simulink model "Model_v13"  (R2019a)
settings: Solver=VariableStepAuto  StartTime=0.0  StopTime=t_sim  MaxStep=1e-3  RelTol=1e-6
values from neighbouring files (symbols this model uses):
  b_wheel = 5e-4    (= 0.0005)    [Parameters.m]    (also in UKFMeasurementFcn.m; UKFTransitionFcn.m)
  H = 0.075    [Parameters.m]    (also in SMC_one_wheel.m; UKFMeasurementFcn.m; UKFTransitionFcn.m)
  J = 0.001    [Parameters.m]    (also in SMC_one_wheel.m = 0.00015; UKFMeasurementFcn.m; UKFTransitionFcn.m)
  Km = 36.9e-3    (= 0.0369)    [Parameters.m]    (also in SMC_one_wheel.m; UKFMeasurementFcn.m; UKFTransitionFcn.m)
  l = l_front + l_rear    (= 0.401)    [Parameters.m]    (also in SMC_one_wheel.m; UKFMeasurementFcn.m; UKFTransitionFcn.m)
  l_front = 0.1968    [Parameters.m]    (also in SMC_one_wheel.m; UKFMeasurementFcn.m; UKFTransitionFcn.m)
  l_rear = 0.2042    [Parameters.m]    (also in SMC_one_wheel.m; UKFMeasurementFcn.m; UKFTransitionFcn.m)
  Lm = 0.463e-3    (= 0.000463)    [Parameters.m]    (also in SMC_one_wheel.m; UKFMeasurementFcn.m; UKFTransitionFcn.m)
  M = 3.832    [Parameters.m]    (also in SMC_one_wheel.m = 0.958; UKFMeasurementFcn.m; UKFTransitionFcn.m)
  R = 0.055    [Parameters.m]    (also in SMC_one_wheel.m; UKFMeasurementFcn.m; UKFTransitionFcn.m; slip_rate.m = args(3))
  Rm = 0.608    [Parameters.m]    (also in SMC_one_wheel.m; UKFMeasurementFcn.m; UKFTransitionFcn.m)
  t_dec = 5    [Parameters.m]
  V_0 = 1    [Parameters.m]
  V_max = 24    [Parameters.m]
  W = M*g    (= 37.59192)    [Parameters.m]    (also in SMC_one_wheel.m = 9.39798; UKFMeasurementFcn.m; UKFTransitionFcn.m)
  w_0 = (1-slip)*V_0/R    (= 18.1818181818)    [Parameters.m]    (also in SMC_one_wheel.m = 90.9090909091)
  WheelSS_A = [-b_wheel/J, Km/J, 0, 0 ... (first row only)    [Parameters.m]
  WheelSS_B = [-R/J, 0, 0, 0 ... (first row only)    [Parameters.m]
  WheelSS_C = [1, 0, 0, 0 ... (first row only)    [Parameters.m]
  WheelSS_D = [0, 0, 0, 0 ... (first row only)    [Parameters.m]
  WheelSS_ICs = [w_0, 0, w_0, 0]    [Parameters.m]
undefined symbols (not defined in the file or in its folder): Discrete, Time
libraries: simulink x11, eeGeneralControl x2, ctrlSharedLib x2
settings Model: Creator=Iansweeney  LastModifiedBy=Iansweeney
settings DataIOCC: ReturnWorkspaceOutputs=off
settings DebuggingCC: UnderSpecifiedDimensionMsg=warning  ArithmeticOperatorsInVariantConditions=warning

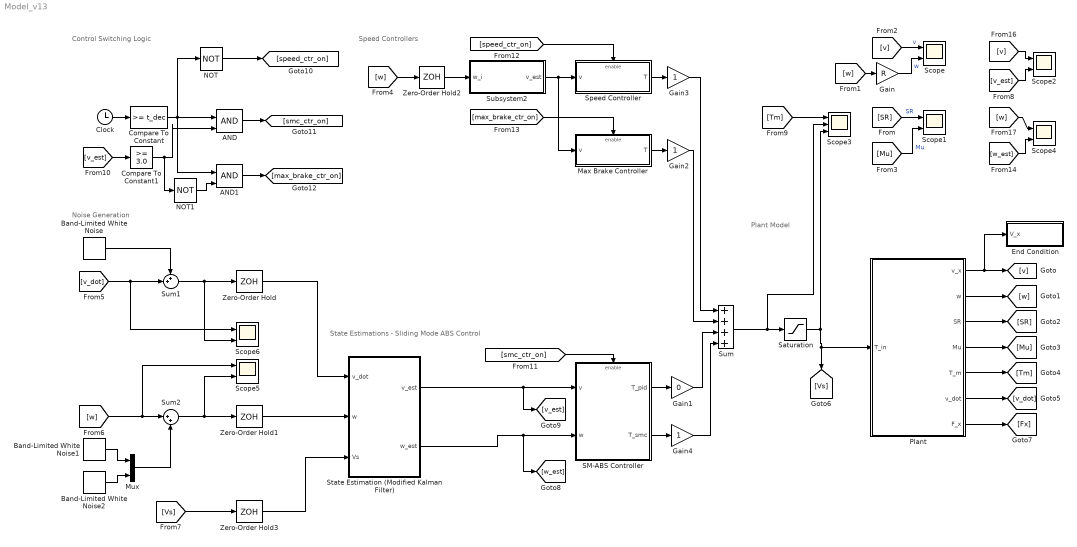
== system Model_v13 ==
  note: State Estimations - Sliding Mode ABS Control
  note: Noise Generation
  note: Speed Controllers
  note: Plant Model
  note: Control Switching Logic
  AND : Logic  IconShape=distinctive  AllPortsSameDT=off  OutDataTypeStr=boolean
  AND1 : Logic  IconShape=distinctive  AllPortsSameDT=off  OutDataTypeStr=boolean
  Band-Limited White Noise : simulink/Sources/Band-Limited White Noise  Cov=[0.001]  Ts=0.001  seed=[23341]
  Band-Limited White Noise1 : simulink/Sources/Band-Limited White Noise  Cov=[0.01]  Ts=0.001  seed=[11111]
  Band-Limited White Noise2 : simulink/Sources/Band-Limited White Noise  Cov=[0.01]  Ts=0.001  seed=[22222]
  Clock : Clock
  Compare To Constant : simulink/Logic and Bit Operations/Compare To Constant  relop=>=  const=t_dec  OutDataTypeStr=boolean
  Compare To Constant1 : simulink/Logic and Bit Operations/Compare To Constant  relop=>=  const=3.0  OutDataTypeStr=boolean
  End Condition : Subsystem
  Gain : Gain  Gain=R
  Gain1 : Gain  Gain=0
  Gain2 : Gain
  Gain3 : Gain
  Gain4 : Gain
  Max Brake Controller : Subsystem
  Mux : Mux  Inputs=2
  NOT : Logic  Operator=NOT  IconShape=distinctive  AllPortsSameDT=off  OutDataTypeStr=boolean
  NOT1 : Logic  Operator=NOT  IconShape=distinctive  AllPortsSameDT=off  OutDataTypeStr=boolean
  Plant : Subsystem
  SM-ABS Controller : Subsystem  TreatAsAtomicUnit=on
  Saturation : Saturate  UpperLimit=V_max  LowerLimit=-V_max
  Scope{,1..2,4..6} (6 alike) : Scope  NumInputPorts=2
  Scope3 : Scope  NumInputPorts=3
  Speed Controller : Subsystem
  State Estimation (Modified Kalman Filter) : Subsystem
  Subsystem2 : Subsystem
  Sum : Sum  Inputs=++++
  Sum1 : Sum  Inputs=++|
  Sum2 : Sum  Inputs=|++
  Zero-Order Hold{,1..3} (4 alike) : ZeroOrderHold  SampleTime=0.01
  wires:
  Plant/1(v_x) -> End Condition/1(V_x), [v]
  Plant/2(w) -> [w]
  Plant/3(SR) -> [SR]
  Plant/4(Mu) -> [Mu]
  Gain/1 -> Scope/2  "w"
  [SR] -> Scope1/1  "SR"
  [w] -> Gain/1
  [v] -> Scope/1  "v"
  [Mu] -> Scope1/2  "Mu"
  Saturation/1 -> Scope3/3, Plant/1(T_in), [Vs]
  Sum/1 -> Scope3/2, Saturation/1
  Plant/5(T_m) -> [Tm]
  [Tm] -> Scope3/1
  SM-ABS Controller/1(T_pid) -> Gain1/1
  Gain1/1 -> Sum/3
  Speed Controller/1(T) -> Gain3/1
  Gain3/1 -> Sum/1
  SM-ABS Controller/2(T_smc) -> Gain4/1
  Gain4/1 -> Sum/4
  Plant/6(v_dot) -> [v_dot]
  Subsystem2/1(v_est) -> Max Brake Controller/1(v), Speed Controller/1(v)
  [w] -> Zero-Order Hold2/1
  Zero-Order Hold2/1 -> Subsystem2/1(w_i)
  Zero-Order Hold/1 -> State Estimation (Modified Kalman Filter)/1(v_dot)
  [Vs] -> Zero-Order Hold3/1
  Zero-Order Hold3/1 -> State Estimation (Modified Kalman Filter)/3(Vs)
  Zero-Order Hold1/1 -> State Estimation (Modified Kalman Filter)/2(w)
  State Estimation (Modified Kalman Filter)/1(v_est) -> [v_est], SM-ABS Controller/1(v)
  Plant/7(F_x) -> [Fx]
  State Estimation (Modified Kalman Filter)/2(w_est) -> [w_est], SM-ABS Controller/2(w)
  [v_est] -> Scope2/2
  [v] -> Scope2/1
  [w] -> Scope4/1
  [w_est] -> Scope4/2
  Band-Limited White Noise/1 -> Sum1/1
  Band-Limited White Noise1/1 -> Mux/1
  Mux/1 -> Sum2/2
  [w] -> Scope5/1, Sum2/1
  Sum2/1 -> Scope5/2, Zero-Order Hold1/1
  [v_dot] -> Scope6/1, Sum1/2
  Sum1/1 -> Scope6/2, Zero-Order Hold/1
  Clock/1 -> Compare To Constant/1
  [v_est] -> Compare To Constant1/1
  AND/1 -> [smc_ctr_on]
  Compare To Constant/1 -> AND1/1, NOT/1, AND/1
  Compare To Constant1/1 -> NOT1/1, AND/2
  [smc_ctr_on] -> SM-ABS Controller/Enable
  NOT/1 -> [speed_ctr_on]
  [speed_ctr_on] -> Speed Controller/Enable
  NOT1/1 -> AND1/2
  AND1/1 -> [max_brake_ctr_on]
  Gain2/1 -> Sum/2
  Max Brake Controller/1(T) -> Gain2/1
  [max_brake_ctr_on] -> Max Brake Controller/Enable
  Band-Limited White Noise2/1 -> Mux/2

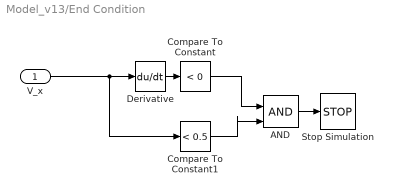
== system Model_v13/End Condition ==
  V_x : Inport
  AND : Logic  IconShape=distinctive  AllPortsSameDT=off  OutDataTypeStr=boolean
  Compare To Constant : simulink/Logic and Bit Operations/Compare To Constant  relop=<  const=0  OutDataTypeStr=boolean
  Compare To Constant1 : simulink/Logic and Bit Operations/Compare To Constant  relop=<  const=0.5  OutDataTypeStr=boolean
  Derivative : Derivative
  Stop Simulation : Stop
  wires:
  AND/1 -> Stop Simulation/1
  Derivative/1 -> Compare To Constant/1
  Compare To Constant/1 -> AND/1
  Compare To Constant1/1 -> AND/2
  V_x/1 -> Compare To Constant1/1, Derivative/1

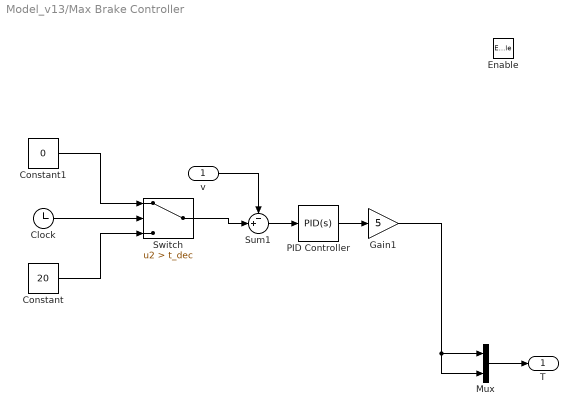
== system Model_v13/Max Brake Controller ==
  v : Inport
  Enable : EnablePort
  Clock : Clock
  Constant : Constant  Value=20
  Constant1 : Constant  Value=0
  Gain1 : Gain  Gain=5
  Mux : Mux  Inputs=2
  PID Controller : simulink/Continuous/PID Controller  Controller=PID  Form=Parallel  TimeDomain=Continuous-time  SampleTime=-1  IntegratorMethod=Forward Euler  FilterMethod=Forward Euler  ControllerParametersSource=internal  P=1  I=0  D=0  UseFilter=on  N=100  TunerSelectOption=Transfer Function Based (PID Tuner App)  InitialConditionSource=internal  InitialConditionForIntegrator=0  InitialConditionForFilter=0  DifferentiatorICPrevScaledInput=0  ExternalReset=none  TrackingMode=off  Kt=1  LimitOutput=off  UpperSaturationLimit=inf  LowerSaturationLimit=-inf  LinearizeAsGain=on  AntiWindupMode=none  Kb=1  POutMin=[]  POutMax=[]  IOutMin=[]  IOutMax=[]  DOutMin=[]  DOutMax=[]  NOutMin=[]  NOutMax=[]  SumOutMin=[]  SumOutMax=[]  SaturationOutMin=[]  SaturationOutMax=[]  PParamMin=[]  PParamMax=[]  IParamMin=[]  IParamMax=[]  DParamMin=[]  DParamMax=[]  NParamMin=[]  NParamMax=[]  KbParamMin=[]  KbParamMax=[]  KtParamMin=[]  KtParamMax=[]  KbOutMin=[]  KbOutMax=[]  KtOutMin=[]  KtOutMax=[]  IntegratorOutMin=[]  IntegratorOutMax=[]  FilterOutMin=[]  FilterOutMax=[]  SumI1OutMin=[]  SumI1OutMax=[]  SumI2OutMin=[]  SumI2OutMax=[]  SumI3OutMin=[]  SumI3OutMax=[]  SumI4OutMin=[]  SumI4OutMax=[]  SumDOutMin=[]  SumDOutMax=[]  DifferentiatorOutMin=[]  DifferentiatorOutMax=[]  FilterDiffOutCoefMin=[]  FilterDiffOutCoefMax=[]  ReciprocalOutMin=[]  ReciprocalOutMax=[]  SumDenOutMin=[]  SumDenOutMax=[]  SumNumOutMin=[]  SumNumOutMax=[]  DivideOutMin=[]  DivideOutMax=[]  IntegratorContinuousStateAttributes=''  IntegratorStateMustResolveToSignalObject=off  IntegratorRTWStateStorageClass=Auto  FilterContinuousStateAttributes=''  FilterStateMustResolveToSignalObject=off  FilterRTWStateStorageClass=Auto  ParallelPVariant=InternalParameters  IdealPVariant=Disabled  IVariant=InternalParameters  DVariant=InternalParameters  IntegratorVariant=Continuous  SatVariant=Disabled  AWVariant=Passthrough  PCopyVariant=Disabled  TRVariant=Disabled  FdbkBlocksVariant=Forward  IdealPFdbkVariant=Disabled  SatFdbkVariant=Disabled  DerivativeFilterVariant=ContFilter  NVariant=InternalParameters  NCopyVariant=Disabled  FilterICVariant=InternalICsFilter  IntegratorICVariant=InternalICs  ExternalResetVariant=Disabled  TRSumVariant=Passthrough  SumFdbkVariant=Disabled  SumVariant=Sum_PID
  Sum1 : Sum  Inputs=-+|
  Switch : Switch  Criteria=u2 > Threshold  Threshold=t_dec
  T : Outport  OutputWhenDisabled=reset  InitialOutput=[0, 0]
  wires:
  PID Controller/1 -> Gain1/1
  Switch/1 -> Sum1/2
  Sum1/1 -> PID Controller/1
  Mux/1 -> T/1
  Gain1/1 -> Mux/2, Mux/1
  v/1 -> Sum1/1
  Constant/1 -> Switch/3
  Constant1/1 -> Switch/1
  Clock/1 -> Switch/2

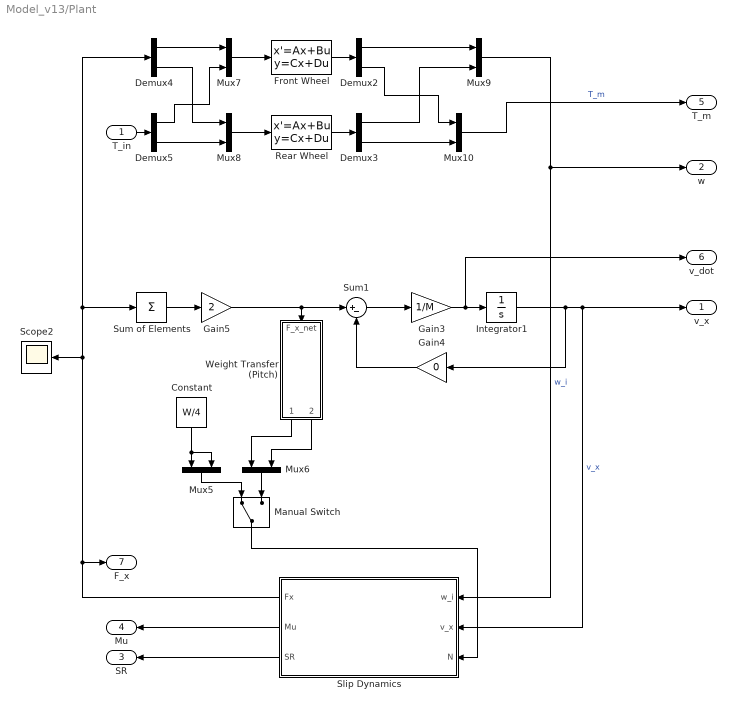
== system Model_v13/Plant ==
  T_in : Inport
  Constant : Constant  Value=W/4
  Demux{2..5} (4 alike) : Demux  Outputs=2
  Front Wheel : StateSpace  A=[-b_wheel/J, Km/J; -Km/J, -Rm/Lm]  B=[-R/J, 0; 0, 1/Lm]  C=[1, 0; 0, Km]  D=[0, 0; 0, 0]  InitialCondition=[w_0, 0]
  Gain3 : Gain  Gain=1/M
  Gain4 : Gain  Gain=0
  Gain5 : Gain  Gain=2
  Integrator1 : Integrator  InitialCondition=V_0
  Manual Switch : ManualSwitch
  Mux{5..10} (6 alike) : Mux  Inputs=2
  Rear Wheel : StateSpace  A=[-b_wheel/J, Km/J; -Km/J, -Rm/Lm]  B=[-R/J, 0; 0, 1/Lm]  C=[1, 0; 0, Km]  D=[0, 0; 0, 0]  InitialCondition=[w_0, 0]
  Scope2 : Scope
  Slip Dynamics : Subsystem
  Sum of Elements : Sum  Inputs=+
  Sum1 : Sum  Inputs=|+-
  Weight Transfer (Pitch) : Subsystem
  v_x : Outport
  w : Outport  Port=2
  SR : Outport  Port=3
  Mu : Outport  Port=4
  T_m : Outport  Port=5
  v_dot : Outport  Port=6
  F_x : Outport  Port=7
  wires:
  Weight Transfer (Pitch)/1(F_z_front) -> Mux6/1
  Weight Transfer (Pitch)/2(F_z_rear) -> Mux6/2
  Gain3/1 -> v_dot/1, Integrator1/1
  Mux5/1 -> Manual Switch/1
  Gain4/1 -> Sum1/2
  T_in/1 -> Demux5/1
  Sum1/1 -> Gain3/1
  Mux6/1 -> Manual Switch/2
  Constant/1 -> Mux5/2, Mux5/1
  Mux9/1 -> w/1, Slip Dynamics/1(w_i)  "w_i"
  Gain5/1 -> Weight Transfer (Pitch)/1(F_x_net), Sum1/1
  Sum of Elements/1 -> Gain5/1
  Integrator1/1 -> Gain4/1, Slip Dynamics/2(v_x), v_x/1  "v_x"
  Mux7/1 -> Front Wheel/1
  Front Wheel/1 -> Demux2/1
  Demux2/1 -> Mux9/1
  Mux8/1 -> Rear Wheel/1
  Rear Wheel/1 -> Demux3/1
  Demux3/1 -> Mux9/2
  Demux4/1 -> Mux7/1
  Demux4/2 -> Mux8/1
  Demux5/1 -> Mux7/2
  Demux5/2 -> Mux8/2
  Demux3/2 -> Mux10/2
  Demux2/2 -> Mux10/1
  Mux10/1 -> T_m/1  "T_m"
  Slip Dynamics/1(Fx) -> F_x/1, Demux4/1, Sum of Elements/1, Scope2/1
  Manual Switch/1 -> Slip Dynamics/3(N)
  Slip Dynamics/2(Mu) -> Mu/1
  Slip Dynamics/3(SR) -> SR/1

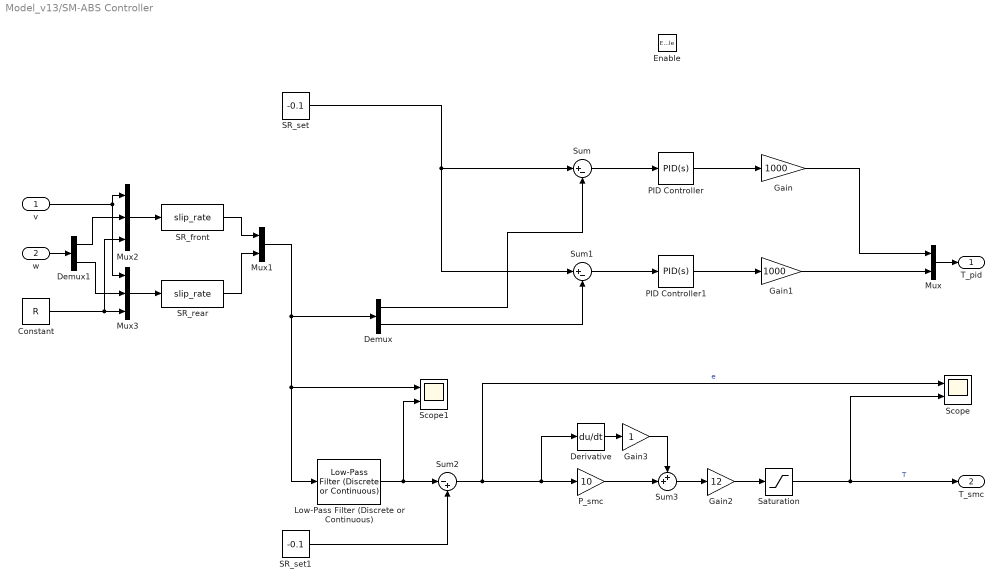
== system Model_v13/SM-ABS Controller ==
  v : Inport
  w : Inport  Port=2
  Enable : EnablePort
  Constant : Constant  Value=R
  Demux : Demux  Outputs=2
  Demux1 : Demux  Outputs=2
  Derivative : Derivative
  Gain : Gain  Gain=1000
  Gain1 : Gain  Gain=1000
  Gain2 : Gain  Gain=12
  Gain3 : Gain
  Low-Pass Filter (Discrete or Continuous) : eeGeneralControl/Low-Pass Filter (Discrete or Continuous)  K=1  T=0.05  B=inf  A=-inf  Ts=-1
      settings: SourceProductName=Simscape Electrical
  Mux : Mux  Inputs=2
  Mux1 : Mux  Inputs=2
  Mux2 : Mux  Inputs=3
  Mux3 : Mux  Inputs=3
  PID Controller : simulink/Continuous/PID Controller  Controller=PID  Form=Parallel  TimeDomain=Continuous-time  SampleTime=-1  IntegratorMethod=Forward Euler  FilterMethod=Forward Euler  ControllerParametersSource=internal  P=1  I=1  D=0  UseFilter=on  N=100  TunerSelectOption=Transfer Function Based (PID Tuner App)  InitialConditionSource=internal  InitialConditionForIntegrator=0  InitialConditionForFilter=0  DifferentiatorICPrevScaledInput=0  ExternalReset=none  TrackingMode=off  Kt=1  LimitOutput=off  UpperSaturationLimit=inf  LowerSaturationLimit=-inf  LinearizeAsGain=on  AntiWindupMode=none  Kb=1  POutMin=[]  POutMax=[]  IOutMin=[]  IOutMax=[]  DOutMin=[]  DOutMax=[]  NOutMin=[]  NOutMax=[]  SumOutMin=[]  SumOutMax=[]  SaturationOutMin=[]  SaturationOutMax=[]  PParamMin=[]  PParamMax=[]  IParamMin=[]  IParamMax=[]  DParamMin=[]  DParamMax=[]  NParamMin=[]  NParamMax=[]  KbParamMin=[]  KbParamMax=[]  KtParamMin=[]  KtParamMax=[]  KbOutMin=[]  KbOutMax=[]  KtOutMin=[]  KtOutMax=[]  IntegratorOutMin=[]  IntegratorOutMax=[]  FilterOutMin=[]  FilterOutMax=[]  SumI1OutMin=[]  SumI1OutMax=[]  SumI2OutMin=[]  SumI2OutMax=[]  SumI3OutMin=[]  SumI3OutMax=[]  SumI4OutMin=[]  SumI4OutMax=[]  SumDOutMin=[]  SumDOutMax=[]  DifferentiatorOutMin=[]  DifferentiatorOutMax=[]  FilterDiffOutCoefMin=[]  FilterDiffOutCoefMax=[]  ReciprocalOutMin=[]  ReciprocalOutMax=[]  SumDenOutMin=[]  SumDenOutMax=[]  SumNumOutMin=[]  SumNumOutMax=[]  DivideOutMin=[]  DivideOutMax=[]  IntegratorContinuousStateAttributes=''  IntegratorStateMustResolveToSignalObject=off  IntegratorRTWStateStorageClass=Auto  FilterContinuousStateAttributes=''  FilterStateMustResolveToSignalObject=off  FilterRTWStateStorageClass=Auto  ParallelPVariant=InternalParameters  IdealPVariant=Disabled  IVariant=InternalParameters  DVariant=InternalParameters  IntegratorVariant=Continuous  SatVariant=Disabled  AWVariant=Passthrough  PCopyVariant=Disabled  TRVariant=Disabled  FdbkBlocksVariant=Forward  IdealPFdbkVariant=Disabled  SatFdbkVariant=Disabled  DerivativeFilterVariant=ContFilter  NVariant=InternalParameters  NCopyVariant=Disabled  FilterICVariant=InternalICsFilter  IntegratorICVariant=InternalICs  ExternalResetVariant=Disabled  TRSumVariant=Passthrough  SumFdbkVariant=Disabled  SumVariant=Sum_PID
  PID Controller1 : simulink/Continuous/PID Controller  Controller=PID  Form=Parallel  TimeDomain=Continuous-time  SampleTime=-1  IntegratorMethod=Forward Euler  FilterMethod=Forward Euler  ControllerParametersSource=internal  P=1  I=1  D=0  UseFilter=on  N=100  TunerSelectOption=Transfer Function Based (PID Tuner App)  InitialConditionSource=internal  InitialConditionForIntegrator=0  InitialConditionForFilter=0  DifferentiatorICPrevScaledInput=0  ExternalReset=none  TrackingMode=off  Kt=1  LimitOutput=off  UpperSaturationLimit=inf  LowerSaturationLimit=-inf  LinearizeAsGain=on  AntiWindupMode=none  Kb=1  POutMin=[]  POutMax=[]  IOutMin=[]  IOutMax=[]  DOutMin=[]  DOutMax=[]  NOutMin=[]  NOutMax=[]  SumOutMin=[]  SumOutMax=[]  SaturationOutMin=[]  SaturationOutMax=[]  PParamMin=[]  PParamMax=[]  IParamMin=[]  IParamMax=[]  DParamMin=[]  DParamMax=[]  NParamMin=[]  NParamMax=[]  KbParamMin=[]  KbParamMax=[]  KtParamMin=[]  KtParamMax=[]  KbOutMin=[]  KbOutMax=[]  KtOutMin=[]  KtOutMax=[]  IntegratorOutMin=[]  IntegratorOutMax=[]  FilterOutMin=[]  FilterOutMax=[]  SumI1OutMin=[]  SumI1OutMax=[]  SumI2OutMin=[]  SumI2OutMax=[]  SumI3OutMin=[]  SumI3OutMax=[]  SumI4OutMin=[]  SumI4OutMax=[]  SumDOutMin=[]  SumDOutMax=[]  DifferentiatorOutMin=[]  DifferentiatorOutMax=[]  FilterDiffOutCoefMin=[]  FilterDiffOutCoefMax=[]  ReciprocalOutMin=[]  ReciprocalOutMax=[]  SumDenOutMin=[]  SumDenOutMax=[]  SumNumOutMin=[]  SumNumOutMax=[]  DivideOutMin=[]  DivideOutMax=[]  IntegratorContinuousStateAttributes=''  IntegratorStateMustResolveToSignalObject=off  IntegratorRTWStateStorageClass=Auto  FilterContinuousStateAttributes=''  FilterStateMustResolveToSignalObject=off  FilterRTWStateStorageClass=Auto  ParallelPVariant=InternalParameters  IdealPVariant=Disabled  IVariant=InternalParameters  DVariant=InternalParameters  IntegratorVariant=Continuous  SatVariant=Disabled  AWVariant=Passthrough  PCopyVariant=Disabled  TRVariant=Disabled  FdbkBlocksVariant=Forward  IdealPFdbkVariant=Disabled  SatFdbkVariant=Disabled  DerivativeFilterVariant=ContFilter  NVariant=InternalParameters  NCopyVariant=Disabled  FilterICVariant=InternalICsFilter  IntegratorICVariant=InternalICs  ExternalResetVariant=Disabled  TRSumVariant=Passthrough  SumFdbkVariant=Disabled  SumVariant=Sum_PID
  P_smc : Gain  Gain=10
  SR_front : MATLABFcn  MATLABFcn=slip_rate  OutputDimensions=1
  SR_rear : MATLABFcn  MATLABFcn=slip_rate  OutputDimensions=1
  SR_set : Constant  Value=-0.1
  SR_set1 : Constant  Value=-0.1
  Saturation : Saturate  UpperLimit=24  LowerLimit=-24
  Scope : Scope  NumInputPorts=2
  Scope1 : Scope  NumInputPorts=2
  Sum : Sum  Inputs=|+-
  Sum1 : Sum  Inputs=|+-
  Sum2 : Sum  Inputs=|-+
  Sum3 : Sum  Inputs=++|
  T_pid : Outport  OutputWhenDisabled=reset  InitialOutput=[0, 0]
  T_smc : Outport  Port=2
  wires:
  Mux/1 -> T_pid/1
  Sum/1 -> PID Controller/1
  Demux/1 -> Sum/2
  PID Controller/1 -> Gain/1
  Gain/1 -> Mux/1
  Sum1/1 -> PID Controller1/1
  PID Controller1/1 -> Gain1/1
  SR_set/1 -> Sum1/1, Sum/1
  Gain1/1 -> Mux/2
  Demux/2 -> Sum1/2
  SR_set1/1 -> Sum2/2
  Sum2/1 -> Scope/1, P_smc/1, Derivative/1  "e"
  P_smc/1 -> Sum3/2
  Sum3/1 -> Gain2/1
  Gain2/1 -> Saturation/1
  Saturation/1 -> Scope/2, T_smc/1  "T"
  SR_front/1 -> Mux1/1
  SR_rear/1 -> Mux1/2
  Mux3/1 -> SR_rear/1
  Mux2/1 -> SR_front/1
  Demux1/2 -> Mux3/2
  Demux1/1 -> Mux2/2
  v/1 -> Mux3/1, Mux2/1
  Constant/1 -> Mux2/3, Mux3/3
  w/1 -> Demux1/1
  Low-Pass Filter (Discrete or Continuous)/1 -> Scope1/2, Sum2/1
  Mux1/1 -> Demux/1, Low-Pass Filter (Discrete or Continuous)/1, Scope1/1
  Derivative/1 -> Gain3/1
  Gain3/1 -> Sum3/1

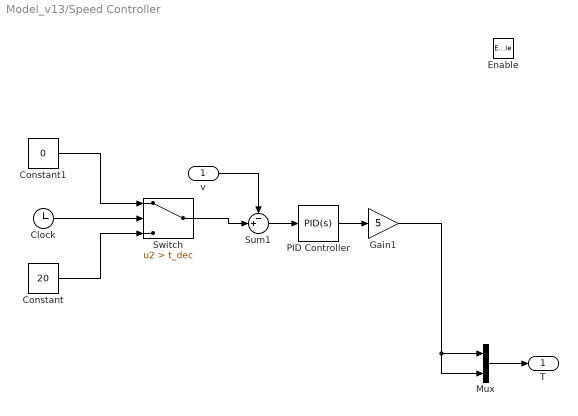
== system Model_v13/Speed Controller ==
  v : Inport
  Enable : EnablePort
  Clock : Clock
  Constant : Constant  Value=20
  Constant1 : Constant  Value=0
  Gain1 : Gain  Gain=5
  Mux : Mux  Inputs=2
  PID Controller : simulink/Continuous/PID Controller  Controller=PID  Form=Parallel  TimeDomain=Continuous-time  SampleTime=-1  IntegratorMethod=Forward Euler  FilterMethod=Forward Euler  ControllerParametersSource=internal  P=1  I=1  D=0  UseFilter=on  N=100  TunerSelectOption=Transfer Function Based (PID Tuner App)  InitialConditionSource=internal  InitialConditionForIntegrator=0  InitialConditionForFilter=0  DifferentiatorICPrevScaledInput=0  ExternalReset=none  TrackingMode=off  Kt=1  LimitOutput=off  UpperSaturationLimit=inf  LowerSaturationLimit=-inf  LinearizeAsGain=on  AntiWindupMode=none  Kb=1  POutMin=[]  POutMax=[]  IOutMin=[]  IOutMax=[]  DOutMin=[]  DOutMax=[]  NOutMin=[]  NOutMax=[]  SumOutMin=[]  SumOutMax=[]  SaturationOutMin=[]  SaturationOutMax=[]  PParamMin=[]  PParamMax=[]  IParamMin=[]  IParamMax=[]  DParamMin=[]  DParamMax=[]  NParamMin=[]  NParamMax=[]  KbParamMin=[]  KbParamMax=[]  KtParamMin=[]  KtParamMax=[]  KbOutMin=[]  KbOutMax=[]  KtOutMin=[]  KtOutMax=[]  IntegratorOutMin=[]  IntegratorOutMax=[]  FilterOutMin=[]  FilterOutMax=[]  SumI1OutMin=[]  SumI1OutMax=[]  SumI2OutMin=[]  SumI2OutMax=[]  SumI3OutMin=[]  SumI3OutMax=[]  SumI4OutMin=[]  SumI4OutMax=[]  SumDOutMin=[]  SumDOutMax=[]  DifferentiatorOutMin=[]  DifferentiatorOutMax=[]  FilterDiffOutCoefMin=[]  FilterDiffOutCoefMax=[]  ReciprocalOutMin=[]  ReciprocalOutMax=[]  SumDenOutMin=[]  SumDenOutMax=[]  SumNumOutMin=[]  SumNumOutMax=[]  DivideOutMin=[]  DivideOutMax=[]  IntegratorContinuousStateAttributes=''  IntegratorStateMustResolveToSignalObject=off  IntegratorRTWStateStorageClass=Auto  FilterContinuousStateAttributes=''  FilterStateMustResolveToSignalObject=off  FilterRTWStateStorageClass=Auto  ParallelPVariant=InternalParameters  IdealPVariant=Disabled  IVariant=InternalParameters  DVariant=InternalParameters  IntegratorVariant=Continuous  SatVariant=Disabled  AWVariant=Passthrough  PCopyVariant=Disabled  TRVariant=Disabled  FdbkBlocksVariant=Forward  IdealPFdbkVariant=Disabled  SatFdbkVariant=Disabled  DerivativeFilterVariant=ContFilter  NVariant=InternalParameters  NCopyVariant=Disabled  FilterICVariant=InternalICsFilter  IntegratorICVariant=InternalICs  ExternalResetVariant=Disabled  TRSumVariant=Passthrough  SumFdbkVariant=Disabled  SumVariant=Sum_PID
  Sum1 : Sum  Inputs=-+|
  Switch : Switch  Criteria=u2 > Threshold  Threshold=t_dec
  T : Outport  OutputWhenDisabled=reset  InitialOutput=[0, 0]
  wires:
  PID Controller/1 -> Gain1/1
  Switch/1 -> Sum1/2
  Sum1/1 -> PID Controller/1
  Mux/1 -> T/1
  Gain1/1 -> Mux/2, Mux/1
  v/1 -> Sum1/1
  Constant/1 -> Switch/3
  Constant1/1 -> Switch/1
  Clock/1 -> Switch/2

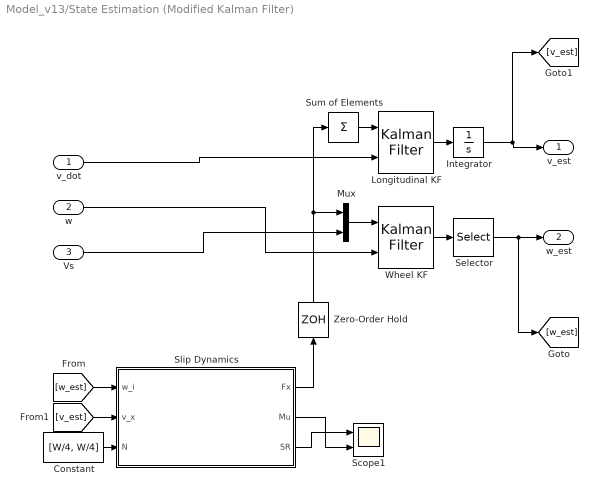
== system Model_v13/State Estimation (Modified Kalman Filter) ==
  v_dot : Inport
  w : Inport  Port=2
  Vs : Inport  Port=3
  Constant : Constant  Value=[W/4, W/4]
  Integrator : Integrator  InitialCondition=V_0
  Longitudinal KF : ctrlSharedLib/Kalman Filter  TimeDomain=Discrete-Time  UseCurrentEstimator=on  ModelSource=Individual A, B, C, D matrices  ModelSourceVariable=ss(0.95,1,1,0,1)  A=0  B=[2/M]  C=0  D=[2/M]  NumberOfStates=1  NumberOfInputs=1  NumberOfOutputs=1  InitialEstimateSource=Dialog  X0=V_0  P0=10  UseK=off  UseGH=off  NumberOfProcessNoiseInputs=1  G=1  TimeInvariantG=on  H=0  TimeInvariantH=on  Q=0.05  TimeInvariantQ=on  R=1  TimeInvariantR=on  N=0  TimeInvariantN=on  AddInputPort=on  AddEnablePort=off  OutputEstimatedY=off  OutputP=off  Ts=-1
      settings: SourceProductBaseCode=CT
  Mux : Mux  Inputs=2
  Scope1 : Scope  NumInputPorts=2
  Selector : Selector  InputPortWidth=4  IndexOptions=Index vector (dialog)  Indices=[1 3]  OutputSizes=1
  Slip Dynamics : Subsystem
  Sum of Elements : Sum  Inputs=+
  Wheel KF : ctrlSharedLib/Kalman Filter  TimeDomain=Discrete-Time  UseCurrentEstimator=on  ModelSource=Individual A, B, C, D matrices  ModelSourceVariable=ss(0.95,1,1,0,1)  A=WheelSS_A  B=WheelSS_B  C=WheelSS_C  D=WheelSS_D  NumberOfStates=1  NumberOfInputs=1  NumberOfOutputs=1  InitialEstimateSource=Dialog  X0=WheelSS_ICs  P0=10  UseK=off  UseGH=off  NumberOfProcessNoiseInputs=1  G=1  TimeInvariantG=on  H=0  TimeInvariantH=on  Q=0.05  TimeInvariantQ=on  R=1  TimeInvariantR=on  N=0  TimeInvariantN=on  AddInputPort=on  AddEnablePort=off  OutputEstimatedY=off  OutputP=off  Ts=-1
      settings: SourceProductBaseCode=CT
  Zero-Order Hold : ZeroOrderHold  SampleTime=0.01
  v_est : Outport
  w_est : Outport  Port=2
  wires:
  Constant/1 -> Slip Dynamics/3(N)
  Wheel KF/1 -> Selector/1
  Selector/1 -> w_est/1, [w_est]
  Mux/1 -> Wheel KF/1
  Vs/1 -> Mux/2
  [w_est] -> Slip Dynamics/1(w_i)
  [v_est] -> Slip Dynamics/2(v_x)
  w/1 -> Wheel KF/2
  Slip Dynamics/2(Mu) -> Scope1/2
  Slip Dynamics/3(SR) -> Scope1/1
  v_dot/1 -> Longitudinal KF/2
  Sum of Elements/1 -> Longitudinal KF/1
  Longitudinal KF/1 -> Integrator/1
  Integrator/1 -> [v_est], v_est/1
  Slip Dynamics/1(Fx) -> Zero-Order Hold/1
  Zero-Order Hold/1 -> Mux/1, Sum of Elements/1

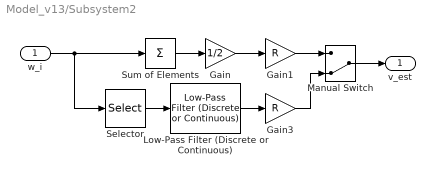
== system Model_v13/Subsystem2 ==
  w_i : Inport
  Gain : Gain  Gain=1/2
  Gain1 : Gain  Gain=R
  Gain3 : Gain  Gain=R
  Low-Pass Filter (Discrete or Continuous) : eeGeneralControl/Low-Pass Filter (Discrete or Continuous)  K=1  T=0.05  B=inf  A=-inf  Ts=-1
      settings: SourceProductName=Simscape Electrical
  Manual Switch : ManualSwitch  CurrentSetting=0
  Selector : Selector  InputPortWidth=2  IndexOptions=Index vector (dialog)  Indices=[1]  OutputSizes=1
  Sum of Elements : Sum  Inputs=+
  v_est : Outport
  wires:
  w_i/1 -> Sum of Elements/1, Selector/1
  Sum of Elements/1 -> Gain/1
  Gain/1 -> Gain1/1
  Gain1/1 -> Manual Switch/1
  Gain3/1 -> Manual Switch/2
  Manual Switch/1 -> v_est/1
  Selector/1 -> Low-Pass Filter (Discrete or Continuous)/1
  Low-Pass Filter (Discrete or Continuous)/1 -> Gain3/1

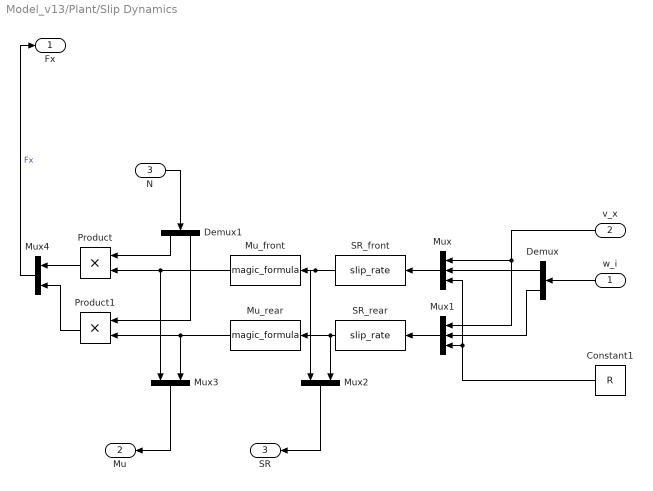
== system Model_v13/Plant/Slip Dynamics ==
  w_i : Inport
  v_x : Inport  Port=2
  N : Inport  Port=3
  Constant1 : Constant  Value=R
  Demux : Demux  Outputs=2
  Demux1 : Demux  Outputs=2
  Mu_front : MATLABFcn  MATLABFcn=magic_formula  OutputDimensions=1
  Mu_rear : MATLABFcn  MATLABFcn=magic_formula  OutputDimensions=1
  Mux : Mux  Inputs=3
  Mux1 : Mux  Inputs=3
  Mux2 : Mux  Inputs=2
  Mux3 : Mux  Inputs=2
  Mux4 : Mux  Inputs=2
  Product : Product
  Product1 : Product
  SR_front : MATLABFcn  MATLABFcn=slip_rate  OutputDimensions=1
  SR_rear : MATLABFcn  MATLABFcn=slip_rate  OutputDimensions=1
  Fx : Outport
  Mu : Outport  Port=2
  SR : Outport  Port=3
  wires:
  Product/1 -> Mux4/1
  Product1/1 -> Mux4/2
  Mux/1 -> SR_front/1
  Mux3/1 -> Mu/1
  Demux/2 -> Mux1/2
  SR_rear/1 -> Mu_rear/1, Mux2/2
  Mu_rear/1 -> Product1/2, Mux3/2
  Constant1/1 -> Mux/3, Mux1/3
  SR_front/1 -> Mux2/1, Mu_front/1
  Mux4/1 -> Fx/1  "Fx"
  v_x/1 -> Mux1/1, Mux/1
  Demux1/2 -> Product1/1
  Mu_front/1 -> Product/2, Mux3/1
  N/1 -> Demux1/1
  Demux/1 -> Mux/2
  Mux1/1 -> SR_rear/1
  w_i/1 -> Demux/1
  Mux2/1 -> SR/1
  Demux1/1 -> Product/1

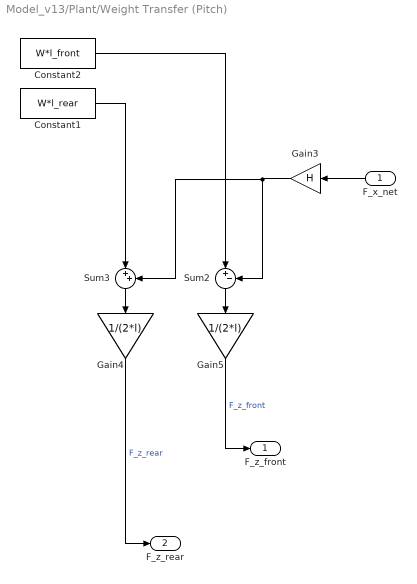
== system Model_v13/Plant/Weight Transfer (Pitch) ==
  F_x_net : Inport
  Constant1 : Constant  Value=W*l_rear
  Constant2 : Constant  Value=W*l_front
  Gain3 : Gain  Gain=H
  Gain4 : Gain  Gain=1/(2*l)
  Gain5 : Gain  Gain=1/(2*l)
  Sum2 : Sum  Inputs=|+-
  Sum3 : Sum  Inputs=|++
  F_z_front : Outport
  F_z_rear : Outport  Port=2
  wires:
  Gain4/1 -> F_z_rear/1  "F_z_rear"
  Gain5/1 -> F_z_front/1  "F_z_front"
  F_x_net/1 -> Gain3/1
  Constant2/1 -> Sum2/1
  Sum3/1 -> Gain4/1
  Constant1/1 -> Sum3/1
  Sum2/1 -> Gain5/1
  Gain3/1 -> Sum3/2, Sum2/2

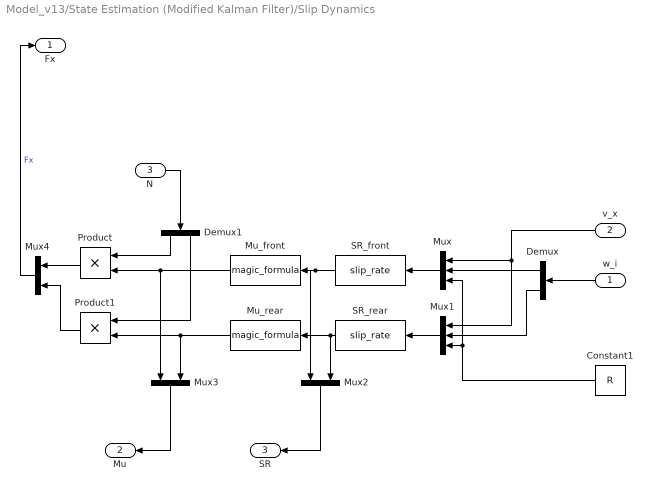
== system Model_v13/State Estimation (Modified Kalman Filter)/Slip Dynamics ==
  w_i : Inport
  v_x : Inport  Port=2
  N : Inport  Port=3
  Constant1 : Constant  Value=R
  Demux : Demux  Outputs=2
  Demux1 : Demux  Outputs=2
  Mu_front : MATLABFcn  MATLABFcn=magic_formula  OutputDimensions=1
  Mu_rear : MATLABFcn  MATLABFcn=magic_formula  OutputDimensions=1
  Mux : Mux  Inputs=3
  Mux1 : Mux  Inputs=3
  Mux2 : Mux  Inputs=2
  Mux3 : Mux  Inputs=2
  Mux4 : Mux  Inputs=2
  Product : Product
  Product1 : Product
  SR_front : MATLABFcn  MATLABFcn=slip_rate  OutputDimensions=1
  SR_rear : MATLABFcn  MATLABFcn=slip_rate  OutputDimensions=1
  Fx : Outport
  Mu : Outport  Port=2
  SR : Outport  Port=3
  wires:
  Product/1 -> Mux4/1
  Product1/1 -> Mux4/2
  Mux/1 -> SR_front/1
  Mux3/1 -> Mu/1
  Demux/2 -> Mux1/2
  SR_rear/1 -> Mu_rear/1, Mux2/2
  Mu_rear/1 -> Product1/2, Mux3/2
  Constant1/1 -> Mux/3, Mux1/3
  SR_front/1 -> Mux2/1, Mu_front/1
  Mux4/1 -> Fx/1  "Fx"
  v_x/1 -> Mux1/1, Mux/1
  Demux1/2 -> Product1/1
  Mu_front/1 -> Product/2, Mux3/1
  N/1 -> Demux1/1
  Demux/1 -> Mux/2
  Mux1/1 -> SR_rear/1
  w_i/1 -> Demux/1
  Mux2/1 -> SR/1
  Demux1/1 -> Product/1
